simulink model "Modelodesimulacion"  (R2015a)
settings: Solver=ode45  StartTime=0.0  StopTime=0.001  RelTol=1e-3
values from neighbouring files (symbols this model uses):
  C = 10e-6    (= 1e-05)    [ejercicio.m]    (also in ejercicio2.m)
  q0 = v0*C    (= 1e-06)    [ejercicio.m]
  R = 10    [ejercicio.m]
  T = R*C    (= 0.0001)    [ejercicio.m]    (also in ejercicio2.m = 7.5e-05)
settings Model: Creator=Daniel Santos  LastModifiedBy=Daniel Santos

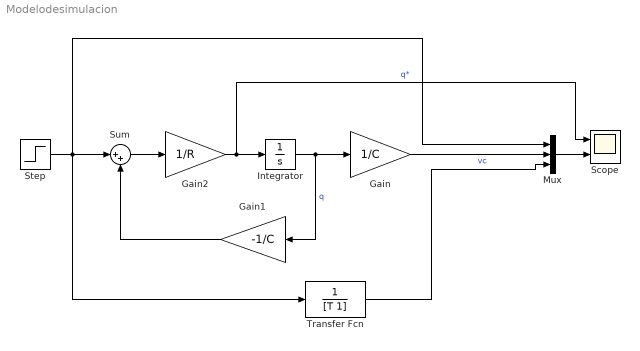
== system Modelodesimulacion ==
  Gain : Gain  Gain=1/C
  Gain1 : Gain  Gain=-1/C
  Gain2 : Gain  Gain=1/R
  Integrator : Integrator  InitialCondition=q0
  Mux : Mux  Inputs=3
  Scope : Scope  NumInputPorts=2
      settings: YMin=-5~-5  YMax=5~5
  Step : Step  Time=0  SampleTime=0
  Sum : Sum  Inputs=|++
  Transfer Fcn : TransferFcn  Denominator=[T 1]
  wires:
  Gain2/1 -> Scope/1, Integrator/1  "q*"
  Integrator/1 -> Gain/1, Gain1/1  "q"
  Gain1/1 -> Sum/2
  Step/1 -> Transfer Fcn/1, Mux/1, Sum/1
  Gain/1 -> Mux/2  "vc"
  Sum/1 -> Gain2/1
  Transfer Fcn/1 -> Mux/3
  Mux/1 -> Scope/2
